simulink model "FOC_PIL_StateMch_top"  (R2026a)
settings: Solver=FixedStepAuto  StopTime=4  FixedStep=6.25e-5
undefined symbols (not defined in the file or in its folder): McInput_Default, McPlant_Params
settings Model: DataDictionary=McData.sldd  Creator=k  LastModifiedBy=k
settings OptimizationCC: UseDivisionForNetSlopeComputation=on  GainParamInheritBuiltInType=on  UseFloatMulNetSlope=on  InlineInvariantSignals=on  NoFixptDivByZeroProtection=on  EfficientFloat2IntCast=on  LifeSpan=1
settings RTWCC: SystemTargetFile=ert.tlc  GenerateReport=on  IncludeHyperlinkInReport=on  GenerateTraceInfo=on  GenerateTraceReport=on  GenerateTraceReportSl=on  GenerateTraceReportSf=on  GenerateTraceReportEml=on  GenerateCodeMetricsReport=on  Description=Embedded Coder
settings ERTTargetCC: GenerateSampleERTMain=on  IncludeMdlTerminateFcn=off  CombineSignalStateStructs=on  SupportContinuousTime=on  SupportNonInlinedSFcns=on

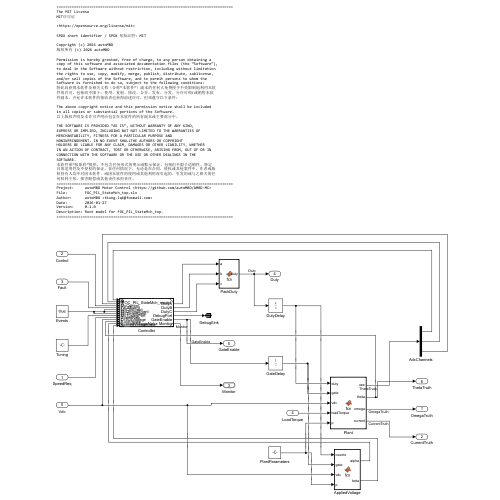
[thumbnail: Simulink's stored preview of the top-level diagram]
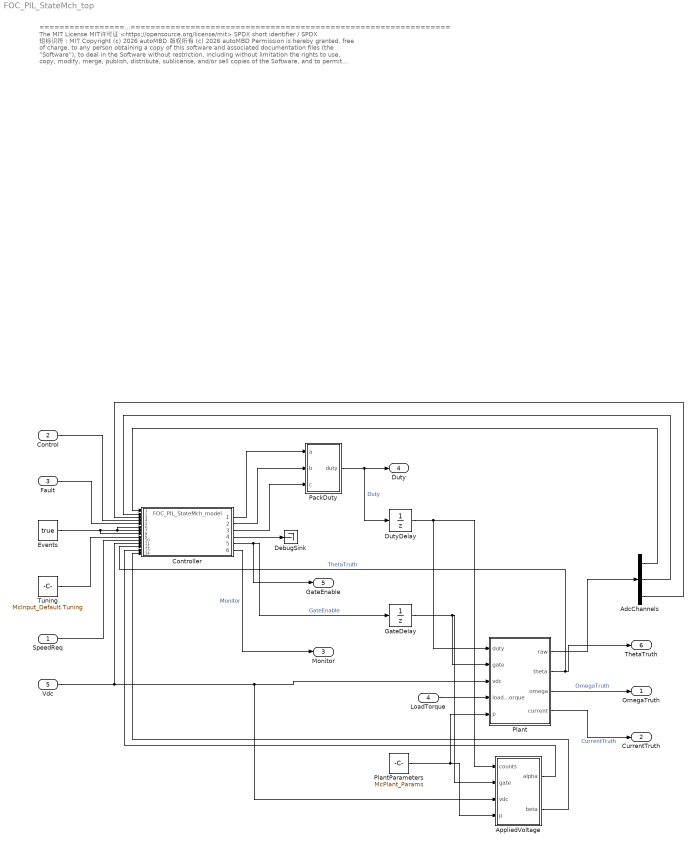
== system FOC_PIL_StateMch_top ==
  note: =================================================================================
      | The MIT License
      | MIT许可证
      |
      | <https://opensource.org/license/mit>
      |
      | SPDX short identifier / SPDX 短标识符：MIT
      |
      | Copyright (c) 2026 autoMBD
      | 版权所有 (c) 2026 autoMBD
      |
      | Permission is hereby granted, free of charge, to any person obtaining a
      | copy of this software and associated documentation files (the “Software”),
      | to deal in the Software without restriction, including without limitation
      | the rights to use, copy, modify, merge, publish, distribute, sublicense,
      | and/or sell copies of the Software, and to permit persons to whom the
      | Software is furnished to do so, subject to the following conditions:
      | 特此向获得本软件及相关文档（合称“本软件”）副本的任何人免费授予不受限制地利用本软
      | 件的许可，包括而不限于：使用、复制、修改、合并、发布、分发、分许可和/或销售本软
      | 件副本，并允许本软件的接收者也获得前述许可，但须遵守以下条件：
      |
      | The above copyright notice and this permission notice shall be included
      | in all copies or substantial portions of the Software.
      | 以上版权声明及本许可声明应包含在本软件的所有副本或主要部分中。
      |
      | THE SOFTWARE IS PROVIDED “AS IS”, WITHOUT WARRANTY OF ANY KIND,
      | EXPRESS OR IMPLIED, INCLUDING BUT NOT LIMITED TO THE WARRANTIES OF
      | MERCHANTABILITY, FITNESS FOR A PARTICULAR PURPOSE AND
      | NONINFRINGEMENT. IN NO EVENT SHALLTHE AUTHORS OR COPYRIGHT
      | HOLDERS BE LIABLE FOR ANY CLAIM, DAMAGES OR OTHER LIABILITY, WHETHER
      | IN AN ACTION OF CONTRACT, TORT OR OTHERWISE, ARISING FROM, OUT OF OR IN
      | CONNECTION WITH THE SOFTWARE OR THE USE OR OTHER DEALINGS IN THE
      | SOFTWARE.
      | 本软件系“按原样”提供，不包含任何形式的明示或默示保证，包括但不限于适销性、特定
      | 目的适用性及不侵权的保证。在任何情况下，无论是在合同、侵权或其他案件中，作者或版
      | 权持有人均不对因本软件、或因本软件的使用或其他利用而引起的、引发的或与之相关的任
      | 何权利主张、损害赔偿或其他责任承担责任。
      | =================================================================================
      | Project:     autoMBD Motor Control <https://github.com/autoMBD/AMBD-MC>
      | File:        FOC_PIL_StateMch_top.slx
      | Author:      autoMBD <tkung.lqk@foxmail.com>
      | Date:        2026-01-27
      | Version:     0.1.0
      | Description: Root model for FOC_PIL_StateMch_top.
      | =================================================================================
  SpeedReq : Inport  OutDataTypeStr=single  SampleTime=6.25e-5
  Control : Inport  Port=2  OutDataTypeStr=uint8  SampleTime=6.25e-5
  Fault : Inport  Port=3  OutDataTypeStr=boolean  SampleTime=6.25e-5
  LoadTorque : Inport  Port=4  OutDataTypeStr=double  SampleTime=6.25e-5
  Vdc : Inport  Port=5  OutDataTypeStr=single  SampleTime=6.25e-5
  AdcChannels : Demux  Outputs=3
  AppliedVoltage : MATLAB Function  TreatAsAtomicUnit=on
  Controller : ModelReference  ModelNameDialog=FOC_PIL_StateMch_model  SimulationMode=Normal  ModelReferenceVersion=1.6
  DebugSink : Terminator
  DutyDelay : UnitDelay  InitialCondition=uint16([32768;32768;32768])  SampleTime=6.25e-5
  Events : Constant  Value=true  OutDataTypeStr=boolean
  GateDelay : UnitDelay  InitialCondition=false  SampleTime=6.25e-5
  PackDuty : MATLAB Function  TreatAsAtomicUnit=on
  Plant : MATLAB Function  TreatAsAtomicUnit=on
  PlantParameters : Constant  Value=McPlant_Params  OutDataTypeStr=Bus: tMcControlParams
  Tuning : Constant  Value=McInput_Default.Tuning  OutDataTypeStr=Bus: tMcTuning
  OmegaTruth : Outport  OutDataTypeStr=single
  CurrentTruth : Outport  Port=2  OutDataTypeStr=single
  Monitor : Outport  Port=3  OutDataTypeStr=Bus: tMcMonitor
  Duty : Outport  Port=4  OutDataTypeStr=uint16
  GateEnable : Outport  Port=5  OutDataTypeStr=boolean
  ThetaTruth : Outport  Port=6  OutDataTypeStr=single
  wires:
  AppliedVoltage/2(beta) -> Controller/14
  AppliedVoltage/1(alpha) -> Controller/13
  Events/1 -> Controller/6, Controller/7, Controller/8
  Controller/4 -> DebugSink/1
  Controller/6 -> Monitor/1  "Monitor"
  Controller/5 -> GateDelay/1, GateEnable/1  "GateEnable"
  PackDuty/1(duty) -> Duty/1, DutyDelay/1  "Duty"
  Plant/4(current) -> CurrentTruth/1  "CurrentTruth"
  Plant/3(omega) -> OmegaTruth/1  "OmegaTruth"
  Plant/2(theta) -> ThetaTruth/1, Controller/12  "ThetaTruth"
  SpeedReq/1 -> Controller/10
  Tuning/1 -> Controller/9
  Fault/1 -> Controller/5
  Control/1 -> Controller/4
  Controller/3 -> PackDuty/3(c)
  AdcChannels/3 -> Controller/3
  Controller/2 -> PackDuty/2(b)
  AdcChannels/2 -> Controller/2
  Controller/1 -> PackDuty/1(a)
  AdcChannels/1 -> Controller/1
  Plant/1(raw) -> AdcChannels/1
  PlantParameters/1 -> Plant/5(p), AppliedVoltage/4(p)
  LoadTorque/1 -> Plant/4(loadTorque)
  Vdc/1 -> AppliedVoltage/3(vdc), Plant/3(vdc), Controller/11
  GateDelay/1 -> AppliedVoltage/2(gate), Plant/2(gate)
  DutyDelay/1 -> Plant/1(duty), AppliedVoltage/1(counts)

== matlab function FOC_PIL_StateMch_top/PackDuty ==
  data: a input; duty output; b input; c input
function duty=fcn(a,b,c)
%#codegen
duty=[a;b;c];
end

== matlab function FOC_PIL_StateMch_top/Plant ==
  data: duty input; raw output; gate input; vdc input; loadTorque input; p input; theta output; omega output; current output
function [raw,theta,omega,current]=fcn(duty,gate,vdc,loadTorque,p)
%#codegen
persistent x
if isempty(x),x=zeros(4,1);end
x=mc.plant_step(x,double(duty)/double(p.PwmPeriod),vdc,loadTorque,gate,p,6.25e-5);
[raw,current,theta,omega]=mc.plant_measure(x,p);
end

== matlab function FOC_PIL_StateMch_top/AppliedVoltage ==
  data: counts input; alpha output; gate input; vdc input; p input; beta output
function [alpha,beta]=fcn(counts,gate,vdc,p)
%#codegen
voltage=mc.applied_voltage(counts,vdc,gate,p.PwmPeriod);
alpha=voltage(1);beta=voltage(2);
end
